simulink library "LiveParts"  (Simulink 8.0)
settings: Solver=ode45  StartTime=0.0  StopTime=10.0  RelTol=1e-3
undefined symbols (not defined in the file): unspecifiedConstant, unspecifiedMatrix
settings Model: Creator=christopher.wipf  LastModifiedBy=christopher.wipf

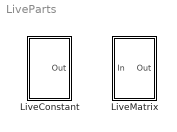
== system LiveParts ==
  LiveConstant : Subsystem  Tag=LiveConstant  mask{K=unspecifiedConstant, chan='unspecifiedChannel'}
      mask prompts: K "Constant"; chan "Channel"
      settings: AttributesFormatString=%<Tag>
      mask Display: disp(K)
  LiveMatrix : Subsystem  Tag=LiveMatrix  mask{M=unspecifiedMatrix, prefix='unspecifiedChannel', firstRow=1, firstCol=1, lastRow=1, lastCol=1}
      mask prompts: M "Matrix"; prefix "Channel prefix"; firstRow "First row"; firstCol "First column"; lastRow "Last row"; lastCol "Last column"
      settings: AttributesFormatString=%<Tag>
      mask Display: disp(M)

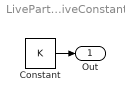
== system LiveParts/LiveConstant ==
  Constant : Constant  Value=K
  Out : Outport
  wires:
  Constant/1 -> Out/1

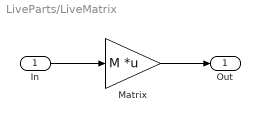
== system LiveParts/LiveMatrix ==
  In : Inport
  Matrix : Gain  Gain=M  Multiplication=Matrix(K*u)
  Out : Outport
  wires:
  In/1 -> Matrix/1
  Matrix/1 -> Out/1
